simulink model "SecRwLtStLgrstInwdOtwdTrgtPosSelc"  (R2018b)
settings: Solver=FixedStepDiscrete  StartTime=0.0  StopTime=10.0  FixedStep=0.01  RelTol=1e-3
undefined symbols (not defined in the file or in its folder): KeSMSw4SAcsMd22SecRwLtStLegrstOtwdInwdPos_Val, KeSMSw4SAcsMd22SecRwLtStLegrstOtwdInwdPosMax_Val, KeSMSw4SAcsMd22SecRwLtStLegrstOtwdInwdPosMin_Val, KeSMSw4SAcsMd26SecRwLtStLegrstOtwdInwdPos_Val, KeSMSw4SAcsMd26SecRwLtStLegrstOtwdInwdPosMax_Val, KeSMSw4SAcsMd26SecRwLtStLegrstOtwdInwdPosMin_Val, KeSMSw4SLegrstCloseMdSecRwLtStLgrstOtwdInwdPos_Val, KeSMSw4SLegrstCloseMdSecRwLtStLgrstOtwdInwdPosMax_Val, KeSMSw4SLegrstCloseMdSecRwLtStLgrstOtwdInwdPosMin_Val, KeSMSw4SLegrstOpenMdSecRwLtStLgrstOtwdInwdPos_Val, KeSMSw4SLegrstOpenMdSecRwLtStLgrstOtwdInwdPosMax_Val, KeSMSw4SLegrstOpenMdSecRwLtStLgrstOtwdInwdPosMin_Val, KeSMSw4sLyingMDSecRwLtStLgrstOtwdInwdPos_160_Val, KeSMSw4sLyingMDSecRwLtStLgrstOtwdInwdPos_165_Val, KeSMSw4sLyingMDSecRwLtStLgrstOtwdInwdPos_170_Val, KeSMSw4sLyingMDSecRwLtStLgrstOtwdInwdPos_175_Val, KeSMSw4sLyingMDSecRwLtStLgrstOtwdInwdPos_180_Val, KeSMSw4sLyingMDSecRwLtStLgrstOtwdInwdPos_Below160_Val, KeSMSw4sLyingMDSecRwLtStLgrstOtwdInwdPos_Over180_Val, KeSMSw4sLyingMDSecRwLtStLgrstOtwdInwdPosMax_160_Val, KeSMSw4sLyingMDSecRwLtStLgrstOtwdInwdPosMax_165_Val, KeSMSw4sLyingMDSecRwLtStLgrstOtwdInwdPosMax_170_Val, KeSMSw4sLyingMDSecRwLtStLgrstOtwdInwdPosMax_175_Val, KeSMSw4sLyingMDSecRwLtStLgrstOtwdInwdPosMax_180_Val, KeSMSw4sLyingMDSecRwLtStLgrstOtwdInwdPosMax_Below160_Val, KeSMSw4sLyingMDSecRwLtStLgrstOtwdInwdPosMax_Over180_Val, KeSMSw4sLyingMDSecRwLtStLgrstOtwdInwdPosMin_160_Val, KeSMSw4sLyingMDSecRwLtStLgrstOtwdInwdPosMin_165_Val, KeSMSw4sLyingMDSecRwLtStLgrstOtwdInwdPosMin_170_Val, KeSMSw4sLyingMDSecRwLtStLgrstOtwdInwdPosMin_175_Val, KeSMSw4sLyingMDSecRwLtStLgrstOtwdInwdPosMin_180_Val, KeSMSw4sLyingMDSecRwLtStLgrstOtwdInwdPosMin_Below160_Val, KeSMSw4sLyingMDSecRwLtStLgrstOtwdInwdPosMin_Over180_Val, KeSMSw4sRecoveryMDSecRwLtStLgrstOtwdInwdPos_160_Val, KeSMSw4sRecoveryMDSecRwLtStLgrstOtwdInwdPos_165_Val, KeSMSw4sRecoveryMDSecRwLtStLgrstOtwdInwdPos_170_Val, KeSMSw4sRecoveryMDSecRwLtStLgrstOtwdInwdPos_175_Val, KeSMSw4sRecoveryMDSecRwLtStLgrstOtwdInwdPos_180_Val, KeSMSw4sRecoveryMDSecRwLtStLgrstOtwdInwdPos_Below160_Val, KeSMSw4sRecoveryMDSecRwLtStLgrstOtwdInwdPos_Over180_Val, KeSMSw4sRecoveryMDSecRwLtStLgrstOtwdInwdPosMax_160_Val, KeSMSw4sRecoveryMDSecRwLtStLgrstOtwdInwdPosMax_165_Val, KeSMSw4sRecoveryMDSecRwLtStLgrstOtwdInwdPosMax_170_Val, KeSMSw4sRecoveryMDSecRwLtStLgrstOtwdInwdPosMax_175_Val, KeSMSw4sRecoveryMDSecRwLtStLgrstOtwdInwdPosMax_180_Val, KeSMSw4sRecoveryMDSecRwLtStLgrstOtwdInwdPosMax_Below160_Val, KeSMSw4sRecoveryMDSecRwLtStLgrstOtwdInwdPosMax_Over180_Val, KeSMSw4sRecoveryMDSecRwLtStLgrstOtwdInwdPosMin_160_Val, KeSMSw4sRecoveryMDSecRwLtStLgrstOtwdInwdPosMin_165_Val, KeSMSw4sRecoveryMDSecRwLtStLgrstOtwdInwdPosMin_170_Val, KeSMSw4sRecoveryMDSecRwLtStLgrstOtwdInwdPosMin_175_Val, KeSMSw4sRecoveryMDSecRwLtStLgrstOtwdInwdPosMin_180_Val, KeSMSw4sRecoveryMDSecRwLtStLgrstOtwdInwdPosMin_Below160_Val, KeSMSw4sRecoveryMDSecRwLtStLgrstOtwdInwdPosMin_Over180_Val, KeSMSw4sVIPMDSecRwLtStLgrstOtwdInwdPos_160_Val, KeSMSw4sVIPMDSecRwLtStLgrstOtwdInwdPos_165_Val, KeSMSw4sVIPMDSecRwLtStLgrstOtwdInwdPos_170_Val, KeSMSw4sVIPMDSecRwLtStLgrstOtwdInwdPos_175_Val, KeSMSw4sVIPMDSecRwLtStLgrstOtwdInwdPos_180_Val, KeSMSw4sVIPMDSecRwLtStLgrstOtwdInwdPos_Below160_Val ... (+36)
libraries: TrgtPosSelcLib x12
(part 2 of 2)

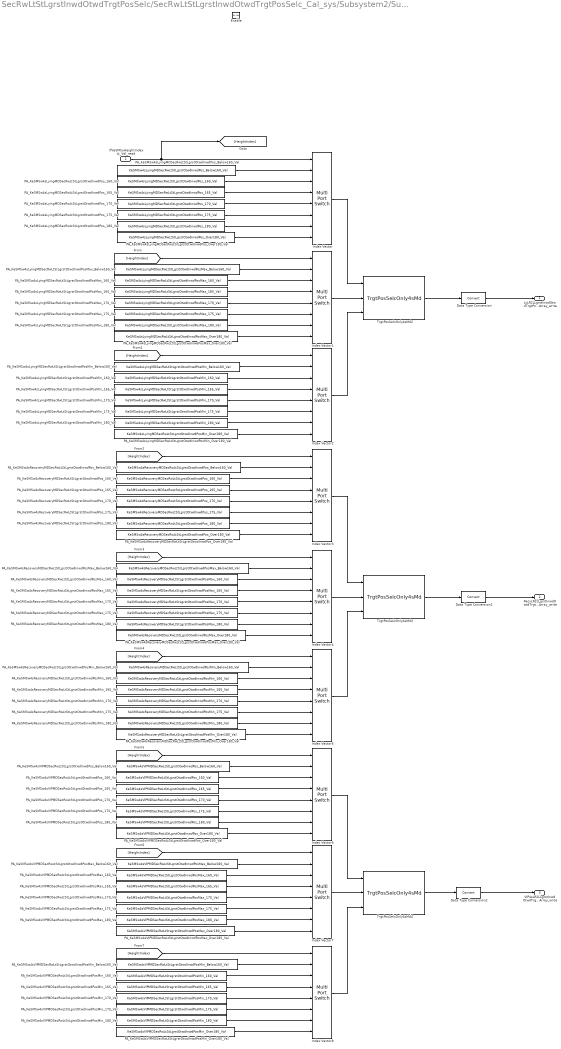
== system SecRwLtStLgrstInwdOtwdTrgtPosSelc/SecRwLtStLgrstInwdOtwdTrgtPosSelc_Cal_sys/Subsystem2/Subsystem1 ==
  IfVeSMSuHeightIndexLt_Val_read : Inport
  Enable : EnablePort
  Data Type Conversion : DataTypeConversion
  Data Type Conversion1 : DataTypeConversion
  Data Type Conversion2 : DataTypeConversion
  Index Vector{,1..8} (9 alike) : MultiPortSwitch  DataPortOrder=Zero-based contiguous  Inputs=7  zeroidx=on
  PA_KeSMSw4sLyingMDSecRwLtStLgrstOtwdInwdPosMax_160_Val : Constant  Value=KeSMSw4sLyingMDSecRwLtStLgrstOtwdInwdPosMax_160_Val
  PA_KeSMSw4sLyingMDSecRwLtStLgrstOtwdInwdPosMax_165_Val : Constant  Value=KeSMSw4sLyingMDSecRwLtStLgrstOtwdInwdPosMax_165_Val
  PA_KeSMSw4sLyingMDSecRwLtStLgrstOtwdInwdPosMax_170_Val : Constant  Value=KeSMSw4sLyingMDSecRwLtStLgrstOtwdInwdPosMax_170_Val
  PA_KeSMSw4sLyingMDSecRwLtStLgrstOtwdInwdPosMax_175_Val : Constant  Value=KeSMSw4sLyingMDSecRwLtStLgrstOtwdInwdPosMax_175_Val
  PA_KeSMSw4sLyingMDSecRwLtStLgrstOtwdInwdPosMax_180_Val : Constant  Value=KeSMSw4sLyingMDSecRwLtStLgrstOtwdInwdPosMax_180_Val
  PA_KeSMSw4sLyingMDSecRwLtStLgrstOtwdInwdPosMax_Below160_Val : Constant  Value=KeSMSw4sLyingMDSecRwLtStLgrstOtwdInwdPosMax_Below160_Val
  PA_KeSMSw4sLyingMDSecRwLtStLgrstOtwdInwdPosMax_Over180_Val : Constant  Value=KeSMSw4sLyingMDSecRwLtStLgrstOtwdInwdPosMax_Over180_Val
  PA_KeSMSw4sLyingMDSecRwLtStLgrstOtwdInwdPosMin_160_Val : Constant  Value=KeSMSw4sLyingMDSecRwLtStLgrstOtwdInwdPosMin_160_Val
  PA_KeSMSw4sLyingMDSecRwLtStLgrstOtwdInwdPosMin_165_Val : Constant  Value=KeSMSw4sLyingMDSecRwLtStLgrstOtwdInwdPosMin_165_Val
  PA_KeSMSw4sLyingMDSecRwLtStLgrstOtwdInwdPosMin_170_Val : Constant  Value=KeSMSw4sLyingMDSecRwLtStLgrstOtwdInwdPosMin_170_Val
  PA_KeSMSw4sLyingMDSecRwLtStLgrstOtwdInwdPosMin_175_Val : Constant  Value=KeSMSw4sLyingMDSecRwLtStLgrstOtwdInwdPosMin_175_Val
  PA_KeSMSw4sLyingMDSecRwLtStLgrstOtwdInwdPosMin_180_Val : Constant  Value=KeSMSw4sLyingMDSecRwLtStLgrstOtwdInwdPosMin_180_Val
  PA_KeSMSw4sLyingMDSecRwLtStLgrstOtwdInwdPosMin_Below160_Val : Constant  Value=KeSMSw4sLyingMDSecRwLtStLgrstOtwdInwdPosMin_Below160_Val
  PA_KeSMSw4sLyingMDSecRwLtStLgrstOtwdInwdPosMin_Over180_Val : Constant  Value=KeSMSw4sLyingMDSecRwLtStLgrstOtwdInwdPosMin_Over180_Val
  PA_KeSMSw4sLyingMDSecRwLtStLgrstOtwdInwdPos_160_Val : Constant  Value=KeSMSw4sLyingMDSecRwLtStLgrstOtwdInwdPos_160_Val
  PA_KeSMSw4sLyingMDSecRwLtStLgrstOtwdInwdPos_165_Val : Constant  Value=KeSMSw4sLyingMDSecRwLtStLgrstOtwdInwdPos_165_Val
  PA_KeSMSw4sLyingMDSecRwLtStLgrstOtwdInwdPos_170_Val : Constant  Value=KeSMSw4sLyingMDSecRwLtStLgrstOtwdInwdPos_170_Val
  PA_KeSMSw4sLyingMDSecRwLtStLgrstOtwdInwdPos_175_Val : Constant  Value=KeSMSw4sLyingMDSecRwLtStLgrstOtwdInwdPos_175_Val
  PA_KeSMSw4sLyingMDSecRwLtStLgrstOtwdInwdPos_180_Val : Constant  Value=KeSMSw4sLyingMDSecRwLtStLgrstOtwdInwdPos_180_Val
  PA_KeSMSw4sLyingMDSecRwLtStLgrstOtwdInwdPos_Below160_Val : Constant  Value=KeSMSw4sLyingMDSecRwLtStLgrstOtwdInwdPos_Below160_Val
  PA_KeSMSw4sLyingMDSecRwLtStLgrstOtwdInwdPos_Over180_Val : Constant  Value=KeSMSw4sLyingMDSecRwLtStLgrstOtwdInwdPos_Over180_Val
  PA_KeSMSw4sRecoveryMDSecRwLtStLgrstOtwdInwdPosMax_160_Val : Constant  Value=KeSMSw4sRecoveryMDSecRwLtStLgrstOtwdInwdPosMax_160_Val
  PA_KeSMSw4sRecoveryMDSecRwLtStLgrstOtwdInwdPosMax_165_Val : Constant  Value=KeSMSw4sRecoveryMDSecRwLtStLgrstOtwdInwdPosMax_165_Val
  PA_KeSMSw4sRecoveryMDSecRwLtStLgrstOtwdInwdPosMax_170_Val : Constant  Value=KeSMSw4sRecoveryMDSecRwLtStLgrstOtwdInwdPosMax_170_Val
  PA_KeSMSw4sRecoveryMDSecRwLtStLgrstOtwdInwdPosMax_175_Val : Constant  Value=KeSMSw4sRecoveryMDSecRwLtStLgrstOtwdInwdPosMax_175_Val
  PA_KeSMSw4sRecoveryMDSecRwLtStLgrstOtwdInwdPosMax_180_Val : Constant  Value=KeSMSw4sRecoveryMDSecRwLtStLgrstOtwdInwdPosMax_180_Val
  PA_KeSMSw4sRecoveryMDSecRwLtStLgrstOtwdInwdPosMax_Below160_Val : Constant  Value=KeSMSw4sRecoveryMDSecRwLtStLgrstOtwdInwdPosMax_Below160_Val
  PA_KeSMSw4sRecoveryMDSecRwLtStLgrstOtwdInwdPosMax_Over180_Val : Constant  Value=KeSMSw4sRecoveryMDSecRwLtStLgrstOtwdInwdPosMax_Over180_Val
  PA_KeSMSw4sRecoveryMDSecRwLtStLgrstOtwdInwdPosMin_160_Val : Constant  Value=KeSMSw4sRecoveryMDSecRwLtStLgrstOtwdInwdPosMin_160_Val
  PA_KeSMSw4sRecoveryMDSecRwLtStLgrstOtwdInwdPosMin_165_Val : Constant  Value=KeSMSw4sRecoveryMDSecRwLtStLgrstOtwdInwdPosMin_165_Val
  PA_KeSMSw4sRecoveryMDSecRwLtStLgrstOtwdInwdPosMin_170_Val : Constant  Value=KeSMSw4sRecoveryMDSecRwLtStLgrstOtwdInwdPosMin_170_Val
  PA_KeSMSw4sRecoveryMDSecRwLtStLgrstOtwdInwdPosMin_175_Val : Constant  Value=KeSMSw4sRecoveryMDSecRwLtStLgrstOtwdInwdPosMin_175_Val
  PA_KeSMSw4sRecoveryMDSecRwLtStLgrstOtwdInwdPosMin_180_Val : Constant  Value=KeSMSw4sRecoveryMDSecRwLtStLgrstOtwdInwdPosMin_180_Val
  PA_KeSMSw4sRecoveryMDSecRwLtStLgrstOtwdInwdPosMin_Below160_Val : Constant  Value=KeSMSw4sRecoveryMDSecRwLtStLgrstOtwdInwdPosMin_Below160_Val
  PA_KeSMSw4sRecoveryMDSecRwLtStLgrstOtwdInwdPosMin_Over180_Val : Constant  Value=KeSMSw4sRecoveryMDSecRwLtStLgrstOtwdInwdPosMin_Over180_Val
  PA_KeSMSw4sRecoveryMDSecRwLtStLgrstOtwdInwdPos_160_Val : Constant  Value=KeSMSw4sRecoveryMDSecRwLtStLgrstOtwdInwdPos_160_Val
  PA_KeSMSw4sRecoveryMDSecRwLtStLgrstOtwdInwdPos_165_Val : Constant  Value=KeSMSw4sRecoveryMDSecRwLtStLgrstOtwdInwdPos_165_Val
  PA_KeSMSw4sRecoveryMDSecRwLtStLgrstOtwdInwdPos_170_Val : Constant  Value=KeSMSw4sRecoveryMDSecRwLtStLgrstOtwdInwdPos_170_Val
  PA_KeSMSw4sRecoveryMDSecRwLtStLgrstOtwdInwdPos_175_Val : Constant  Value=KeSMSw4sRecoveryMDSecRwLtStLgrstOtwdInwdPos_175_Val
  PA_KeSMSw4sRecoveryMDSecRwLtStLgrstOtwdInwdPos_180_Val : Constant  Value=KeSMSw4sRecoveryMDSecRwLtStLgrstOtwdInwdPos_180_Val
  PA_KeSMSw4sRecoveryMDSecRwLtStLgrstOtwdInwdPos_Below160_Val : Constant  Value=KeSMSw4sRecoveryMDSecRwLtStLgrstOtwdInwdPos_Below160_Val
  PA_KeSMSw4sRecoveryMDSecRwLtStLgrstOtwdInwdPos_Over180_Val : Constant  Value=KeSMSw4sRecoveryMDSecRwLtStLgrstOtwdInwdPos_Over180_Val
  PA_KeSMSw4sVIPMDSecRwLtStLgrstOtwdInwdPosMax_160_Val : Constant  Value=KeSMSw4sVIPMDSecRwLtStLgrstOtwdInwdPosMax_160_Val
  PA_KeSMSw4sVIPMDSecRwLtStLgrstOtwdInwdPosMax_165_Val : Constant  Value=KeSMSw4sVIPMDSecRwLtStLgrstOtwdInwdPosMax_165_Val
  PA_KeSMSw4sVIPMDSecRwLtStLgrstOtwdInwdPosMax_170_Val : Constant  Value=KeSMSw4sVIPMDSecRwLtStLgrstOtwdInwdPosMax_170_Val
  PA_KeSMSw4sVIPMDSecRwLtStLgrstOtwdInwdPosMax_175_Val : Constant  Value=KeSMSw4sVIPMDSecRwLtStLgrstOtwdInwdPosMax_175_Val
  PA_KeSMSw4sVIPMDSecRwLtStLgrstOtwdInwdPosMax_180_Val : Constant  Value=KeSMSw4sVIPMDSecRwLtStLgrstOtwdInwdPosMax_180_Val
  PA_KeSMSw4sVIPMDSecRwLtStLgrstOtwdInwdPosMax_Below160_Val : Constant  Value=KeSMSw4sVIPMDSecRwLtStLgrstOtwdInwdPosMax_Below160_Val
  PA_KeSMSw4sVIPMDSecRwLtStLgrstOtwdInwdPosMax_Over180_Val : Constant  Value=KeSMSw4sVIPMDSecRwLtStLgrstOtwdInwdPosMax_Over180_Val
  PA_KeSMSw4sVIPMDSecRwLtStLgrstOtwdInwdPosMin_160_Val : Constant  Value=KeSMSw4sVIPMDSecRwLtStLgrstOtwdInwdPosMin_160_Val
  PA_KeSMSw4sVIPMDSecRwLtStLgrstOtwdInwdPosMin_165_Val : Constant  Value=KeSMSw4sVIPMDSecRwLtStLgrstOtwdInwdPosMin_165_Val
  PA_KeSMSw4sVIPMDSecRwLtStLgrstOtwdInwdPosMin_170_Val : Constant  Value=KeSMSw4sVIPMDSecRwLtStLgrstOtwdInwdPosMin_170_Val
  PA_KeSMSw4sVIPMDSecRwLtStLgrstOtwdInwdPosMin_175_Val : Constant  Value=KeSMSw4sVIPMDSecRwLtStLgrstOtwdInwdPosMin_175_Val
  PA_KeSMSw4sVIPMDSecRwLtStLgrstOtwdInwdPosMin_180_Val : Constant  Value=KeSMSw4sVIPMDSecRwLtStLgrstOtwdInwdPosMin_180_Val
  PA_KeSMSw4sVIPMDSecRwLtStLgrstOtwdInwdPosMin_Below160_Val : Constant  Value=KeSMSw4sVIPMDSecRwLtStLgrstOtwdInwdPosMin_Below160_Val
  PA_KeSMSw4sVIPMDSecRwLtStLgrstOtwdInwdPosMin_Over180_Val : Constant  Value=KeSMSw4sVIPMDSecRwLtStLgrstOtwdInwdPosMin_Over180_Val
  PA_KeSMSw4sVIPMDSecRwLtStLgrstOtwdInwdPos_160_Val : Constant  Value=KeSMSw4sVIPMDSecRwLtStLgrstOtwdInwdPos_160_Val
  PA_KeSMSw4sVIPMDSecRwLtStLgrstOtwdInwdPos_165_Val : Constant  Value=KeSMSw4sVIPMDSecRwLtStLgrstOtwdInwdPos_165_Val
  PA_KeSMSw4sVIPMDSecRwLtStLgrstOtwdInwdPos_170_Val : Constant  Value=KeSMSw4sVIPMDSecRwLtStLgrstOtwdInwdPos_170_Val
  PA_KeSMSw4sVIPMDSecRwLtStLgrstOtwdInwdPos_175_Val : Constant  Value=KeSMSw4sVIPMDSecRwLtStLgrstOtwdInwdPos_175_Val
  PA_KeSMSw4sVIPMDSecRwLtStLgrstOtwdInwdPos_180_Val : Constant  Value=KeSMSw4sVIPMDSecRwLtStLgrstOtwdInwdPos_180_Val
  PA_KeSMSw4sVIPMDSecRwLtStLgrstOtwdInwdPos_Below160_Val : Constant  Value=KeSMSw4sVIPMDSecRwLtStLgrstOtwdInwdPos_Below160_Val
  PA_KeSMSw4sVIPMDSecRwLtStLgrstOtwdInwdPos_Over180_Val : Constant  Value=KeSMSw4sVIPMDSecRwLtStLgrstOtwdInwdPos_Over180_Val
  TrgtPosSelcOnly4sMd2 : TrgtPosSelcLib/TrgtPosSelcOnly4sMd  SystemSampleTime=-1
  TrgtPosSelcOnly4sMd3 : TrgtPosSelcLib/TrgtPosSelcOnly4sMd  SystemSampleTime=-1
  TrgtPosSelcOnly4sMd4 : TrgtPosSelcLib/TrgtPosSelcOnly4sMd  SystemSampleTime=-1
  LyLR2LLgrstInwdOtwdTrgtPosCalib_TrgtPosArray_write : Outport
  RecvLR2LLgrstInwdOtwdTrgtPosCalib_TrgtPosArray_write : Outport  Port=2
  VIP4sLR2LLgrstInwdOtwdTrgtPosCalib_TrgtPosArray_write : Outport  Port=3
  wires:
  PA_KeSMSw4sRecoveryMDSecRwLtStLgrstOtwdInwdPos_Below160_Val/1 -> Index Vector3/2
  PA_KeSMSw4sVIPMDSecRwLtStLgrstOtwdInwdPosMax_180_Val/1 -> Index Vector7/7
  PA_KeSMSw4sLyingMDSecRwLtStLgrstOtwdInwdPos_Below160_Val/1 -> Index Vector/2
  PA_KeSMSw4sRecoveryMDSecRwLtStLgrstOtwdInwdPosMin_175_Val/1 -> Index Vector5/6
  PA_KeSMSw4sVIPMDSecRwLtStLgrstOtwdInwdPosMin_Over180_Val/1 -> Index Vector8/8
  PA_KeSMSw4sVIPMDSecRwLtStLgrstOtwdInwdPosMin_180_Val/1 -> Index Vector8/7
  IfVeSMSuHeightIndexLt_Val_read/1 -> [HeightIndex], Index Vector/1
  PA_KeSMSw4sLyingMDSecRwLtStLgrstOtwdInwdPos_170_Val/1 -> Index Vector/5
  PA_KeSMSw4sRecoveryMDSecRwLtStLgrstOtwdInwdPos_165_Val/1 -> Index Vector3/4
  PA_KeSMSw4sLyingMDSecRwLtStLgrstOtwdInwdPosMin_Below160_Val/1 -> Index Vector2/2
  PA_KeSMSw4sLyingMDSecRwLtStLgrstOtwdInwdPosMax_180_Val/1 -> Index Vector1/7
  PA_KeSMSw4sLyingMDSecRwLtStLgrstOtwdInwdPosMin_175_Val/1 -> Index Vector2/6
  PA_KeSMSw4sRecoveryMDSecRwLtStLgrstOtwdInwdPosMax_175_Val/1 -> Index Vector4/6
  PA_KeSMSw4sRecoveryMDSecRwLtStLgrstOtwdInwdPos_170_Val/1 -> Index Vector3/5
  TrgtPosSelcOnly4sMd3/1 -> Data Type Conversion1/1
  [HeightIndex] -> Index Vector1/1
  PA_KeSMSw4sVIPMDSecRwLtStLgrstOtwdInwdPos_165_Val/1 -> Index Vector6/4
  PA_KeSMSw4sLyingMDSecRwLtStLgrstOtwdInwdPos_180_Val/1 -> Index Vector/7
  PA_KeSMSw4sVIPMDSecRwLtStLgrstOtwdInwdPos_175_Val/1 -> Index Vector6/6
  PA_KeSMSw4sLyingMDSecRwLtStLgrstOtwdInwdPosMax_Over180_Val/1 -> Index Vector1/8
  PA_KeSMSw4sRecoveryMDSecRwLtStLgrstOtwdInwdPosMax_180_Val/1 -> Index Vector4/7
  [HeightIndex] -> Index Vector8/1
  PA_KeSMSw4sLyingMDSecRwLtStLgrstOtwdInwdPosMin_180_Val/1 -> Index Vector2/7
  PA_KeSMSw4sLyingMDSecRwLtStLgrstOtwdInwdPosMax_170_Val/1 -> Index Vector1/5
  PA_KeSMSw4sLyingMDSecRwLtStLgrstOtwdInwdPosMax_Below160_Val/1 -> Index Vector1/2
  PA_KeSMSw4sVIPMDSecRwLtStLgrstOtwdInwdPosMax_Below160_Val/1 -> Index Vector7/2
  PA_KeSMSw4sLyingMDSecRwLtStLgrstOtwdInwdPos_175_Val/1 -> Index Vector/6
  TrgtPosSelcOnly4sMd2/1 -> Data Type Conversion/1
  [HeightIndex] -> Index Vector2/1
  [HeightIndex] -> Index Vector4/1
  PA_KeSMSw4sRecoveryMDSecRwLtStLgrstOtwdInwdPosMax_170_Val/1 -> Index Vector4/5
  PA_KeSMSw4sLyingMDSecRwLtStLgrstOtwdInwdPosMin_Over180_Val/1 -> Index Vector2/8
  PA_KeSMSw4sRecoveryMDSecRwLtStLgrstOtwdInwdPos_180_Val/1 -> Index Vector3/7
  PA_KeSMSw4sRecoveryMDSecRwLtStLgrstOtwdInwdPosMin_180_Val/1 -> Index Vector5/7
  PA_KeSMSw4sLyingMDSecRwLtStLgrstOtwdInwdPosMin_170_Val/1 -> Index Vector2/5
  [HeightIndex] -> Index Vector6/1
  PA_KeSMSw4sLyingMDSecRwLtStLgrstOtwdInwdPos_Over180_Val/1 -> Index Vector/8
  PA_KeSMSw4sVIPMDSecRwLtStLgrstOtwdInwdPosMax_Over180_Val/1 -> Index Vector7/8
  [HeightIndex] -> Index Vector7/1
  PA_KeSMSw4sVIPMDSecRwLtStLgrstOtwdInwdPos_180_Val/1 -> Index Vector6/7
  PA_KeSMSw4sRecoveryMDSecRwLtStLgrstOtwdInwdPosMin_170_Val/1 -> Index Vector5/5
  TrgtPosSelcOnly4sMd4/1 -> Data Type Conversion2/1
  [HeightIndex] -> Index Vector5/1
  PA_KeSMSw4sRecoveryMDSecRwLtStLgrstOtwdInwdPosMax_165_Val/1 -> Index Vector4/4
  PA_KeSMSw4sLyingMDSecRwLtStLgrstOtwdInwdPos_160_Val/1 -> Index Vector/3
  PA_KeSMSw4sRecoveryMDSecRwLtStLgrstOtwdInwdPos_175_Val/1 -> Index Vector3/6
  PA_KeSMSw4sVIPMDSecRwLtStLgrstOtwdInwdPosMax_165_Val/1 -> Index Vector7/4
  PA_KeSMSw4sVIPMDSecRwLtStLgrstOtwdInwdPosMin_165_Val/1 -> Index Vector8/4
  PA_KeSMSw4sLyingMDSecRwLtStLgrstOtwdInwdPosMin_160_Val/1 -> Index Vector2/3
  PA_KeSMSw4sLyingMDSecRwLtStLgrstOtwdInwdPosMin_165_Val/1 -> Index Vector2/4
  PA_KeSMSw4sRecoveryMDSecRwLtStLgrstOtwdInwdPosMax_160_Val/1 -> Index Vector4/3
  [HeightIndex] -> Index Vector3/1
  PA_KeSMSw4sRecoveryMDSecRwLtStLgrstOtwdInwdPos_Over180_Val/1 -> Index Vector3/8
  PA_KeSMSw4sLyingMDSecRwLtStLgrstOtwdInwdPosMax_165_Val/1 -> Index Vector1/4
  PA_KeSMSw4sVIPMDSecRwLtStLgrstOtwdInwdPos_160_Val/1 -> Index Vector6/3
  PA_KeSMSw4sLyingMDSecRwLtStLgrstOtwdInwdPosMax_175_Val/1 -> Index Vector1/6
  PA_KeSMSw4sRecoveryMDSecRwLtStLgrstOtwdInwdPosMin_160_Val/1 -> Index Vector5/3
  PA_KeSMSw4sVIPMDSecRwLtStLgrstOtwdInwdPos_Over180_Val/1 -> Index Vector6/8
  PA_KeSMSw4sLyingMDSecRwLtStLgrstOtwdInwdPos_165_Val/1 -> Index Vector/4
  PA_KeSMSw4sRecoveryMDSecRwLtStLgrstOtwdInwdPosMin_Below160_Val/1 -> Index Vector5/2
  PA_KeSMSw4sRecoveryMDSecRwLtStLgrstOtwdInwdPosMin_Over180_Val/1 -> Index Vector5/8
  PA_KeSMSw4sVIPMDSecRwLtStLgrstOtwdInwdPosMax_175_Val/1 -> Index Vector7/6
  PA_KeSMSw4sVIPMDSecRwLtStLgrstOtwdInwdPosMax_160_Val/1 -> Index Vector7/3
  PA_KeSMSw4sRecoveryMDSecRwLtStLgrstOtwdInwdPos_160_Val/1 -> Index Vector3/3
  PA_KeSMSw4sRecoveryMDSecRwLtStLgrstOtwdInwdPosMin_165_Val/1 -> Index Vector5/4
  PA_KeSMSw4sVIPMDSecRwLtStLgrstOtwdInwdPosMin_160_Val/1 -> Index Vector8/3
  Index Vector/1 -> TrgtPosSelcOnly4sMd2/1
  Index Vector1/1 -> TrgtPosSelcOnly4sMd2/2
  PA_KeSMSw4sVIPMDSecRwLtStLgrstOtwdInwdPos_170_Val/1 -> Index Vector6/5
  Index Vector2/1 -> TrgtPosSelcOnly4sMd2/3
  PA_KeSMSw4sRecoveryMDSecRwLtStLgrstOtwdInwdPosMax_Below160_Val/1 -> Index Vector4/2
  PA_KeSMSw4sVIPMDSecRwLtStLgrstOtwdInwdPosMin_170_Val/1 -> Index Vector8/5
  Index Vector7/1 -> TrgtPosSelcOnly4sMd4/2
  Index Vector5/1 -> TrgtPosSelcOnly4sMd3/3
  Index Vector4/1 -> TrgtPosSelcOnly4sMd3/2
  PA_KeSMSw4sVIPMDSecRwLtStLgrstOtwdInwdPos_Below160_Val/1 -> Index Vector6/2
  PA_KeSMSw4sLyingMDSecRwLtStLgrstOtwdInwdPosMax_160_Val/1 -> Index Vector1/3
  Index Vector6/1 -> TrgtPosSelcOnly4sMd4/1
  PA_KeSMSw4sVIPMDSecRwLtStLgrstOtwdInwdPosMin_Below160_Val/1 -> Index Vector8/2
  PA_KeSMSw4sRecoveryMDSecRwLtStLgrstOtwdInwdPosMax_Over180_Val/1 -> Index Vector4/8
  Index Vector8/1 -> TrgtPosSelcOnly4sMd4/3
  PA_KeSMSw4sVIPMDSecRwLtStLgrstOtwdInwdPosMax_170_Val/1 -> Index Vector7/5
  PA_KeSMSw4sVIPMDSecRwLtStLgrstOtwdInwdPosMin_175_Val/1 -> Index Vector8/6
  Index Vector3/1 -> TrgtPosSelcOnly4sMd3/1
  Data Type Conversion/1 -> LyLR2LLgrstInwdOtwdTrgtPosCalib_TrgtPosArray_write/1
  Data Type Conversion1/1 -> RecvLR2LLgrstInwdOtwdTrgtPosCalib_TrgtPosArray_write/1
  Data Type Conversion2/1 -> VIP4sLR2LLgrstInwdOtwdTrgtPosCalib_TrgtPosArray_write/1

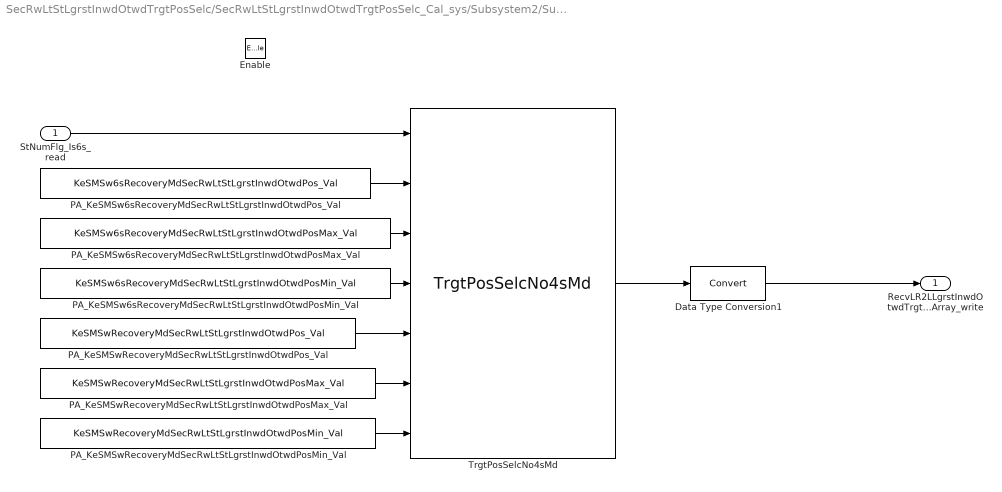
== system SecRwLtStLgrstInwdOtwdTrgtPosSelc/SecRwLtStLgrstInwdOtwdTrgtPosSelc_Cal_sys/Subsystem2/Subsystem2 ==
  StNumFlg_Is6s_read : Inport
  Enable : EnablePort
  Data Type Conversion1 : DataTypeConversion
  PA_KeSMSw6sRecoveryMdSecRwLtStLgrstInwdOtwdPosMax_Val : Constant  Value=KeSMSw6sRecoveryMdSecRwLtStLgrstInwdOtwdPosMax_Val
  PA_KeSMSw6sRecoveryMdSecRwLtStLgrstInwdOtwdPosMin_Val : Constant  Value=KeSMSw6sRecoveryMdSecRwLtStLgrstInwdOtwdPosMin_Val
  PA_KeSMSw6sRecoveryMdSecRwLtStLgrstInwdOtwdPos_Val : Constant  Value=KeSMSw6sRecoveryMdSecRwLtStLgrstInwdOtwdPos_Val
  PA_KeSMSwRecoveryMdSecRwLtStLgrstInwdOtwdPosMax_Val : Constant  Value=KeSMSwRecoveryMdSecRwLtStLgrstInwdOtwdPosMax_Val
  PA_KeSMSwRecoveryMdSecRwLtStLgrstInwdOtwdPosMin_Val : Constant  Value=KeSMSwRecoveryMdSecRwLtStLgrstInwdOtwdPosMin_Val
  PA_KeSMSwRecoveryMdSecRwLtStLgrstInwdOtwdPos_Val : Constant  Value=KeSMSwRecoveryMdSecRwLtStLgrstInwdOtwdPos_Val
  TrgtPosSelcNo4sMd : TrgtPosSelcLib/TrgtPosSelcNo4sMd  SystemSampleTime=-1
  RecvLR2LLgrstInwdOtwdTrgtPosCalib_TrgtPosArray_write : Outport
  wires:
  Data Type Conversion1/1 -> RecvLR2LLgrstInwdOtwdTrgtPosCalib_TrgtPosArray_write/1
  TrgtPosSelcNo4sMd/1 -> Data Type Conversion1/1
  StNumFlg_Is6s_read/1 -> TrgtPosSelcNo4sMd/1
  PA_KeSMSw6sRecoveryMdSecRwLtStLgrstInwdOtwdPos_Val/1 -> TrgtPosSelcNo4sMd/2
  PA_KeSMSw6sRecoveryMdSecRwLtStLgrstInwdOtwdPosMax_Val/1 -> TrgtPosSelcNo4sMd/3
  PA_KeSMSw6sRecoveryMdSecRwLtStLgrstInwdOtwdPosMin_Val/1 -> TrgtPosSelcNo4sMd/4
  PA_KeSMSwRecoveryMdSecRwLtStLgrstInwdOtwdPos_Val/1 -> TrgtPosSelcNo4sMd/5
  PA_KeSMSwRecoveryMdSecRwLtStLgrstInwdOtwdPosMax_Val/1 -> TrgtPosSelcNo4sMd/6
  PA_KeSMSwRecoveryMdSecRwLtStLgrstInwdOtwdPosMin_Val/1 -> TrgtPosSelcNo4sMd/7
